simulink model "esm_wanken"  (R2020b)
settings: Solver=FixedStepAuto  StartTime=simin_radius.time(1,1)  StopTime=simin_radius.time(end,1)-0.01  FixedStep=0.01  RelTol=1e-3  EnableMultiTasking=on
values from neighbouring files (symbols this model uses):
  FZGpars =     [Polo_erweitertesESM.mat]
undefined symbols (not defined in the file or in its folder): magnitude
libraries: simulink x8
settings Model: EnablePacing=on  PacingRate=1000  Creator=Administrator  LastModifiedBy=Laptop 11
settings DataIOCC: ExternalInput=[deltal, v]  SaveFormat=Array  SignalLoggingSaveFormat=ModelDataLogs  ReturnWorkspaceOutputs=off
settings OptimizationCC: ExpressionDepthLimit=2147483647  InitFltsAndDblsToZero=on  LifeSpan=inf
settings DebuggingCC: AlgebraicLoopMsg=none  SaveWithParameterizedLinksMsg=none  UnderspecifiedInitializationDetection=Classic  MergeDetectMultiDrivingBlocksExec=none  SignalResolutionControl=TryResolveAllWithWarning  SolverPrmCheckMsg=warning  MultiTaskDSMMsg=warning  MultiTaskCondExecSysMsg=none  FcnCallInpInsideContextMsg=warning  AllowSymbolicDim=off  StateNameClashWarn=warning  SFUnexpectedBacktrackingDiag=warning  SFNoUnconditionalDefaultTransitionDiag=warning  SFExecutionAtInitializationDiag=none  ArithmeticOperatorsInVariantConditions=warning
settings HardwareCC: ProdBitPerPointer=32  ProdBitPerSizeT=32  ProdBitPerPtrDiffT=32  ProdLargestAtomicFloat=None  ProdIntDivRoundTo=Undefined  ProdEndianess=Unspecified  ProdWordSize=32  ProdHWDeviceType=32-bit Generic
settings ModelReferenceCC: PropagateSignalLabelsOutOfModel=off
settings SFSimCC: SimUseLocalCustomCode=off  CustomCodeUndefinedFunction=UseInterfaceOnly
settings RTWCC: RTWUseLocalCustomCode=off
settings CodeAppCC: StateflowObjectComments=on
settings GRTTargetCC: TargetFcnLib=ansi_tfl_tmw.mat  TargetLangStandard=C89/C90 (ANSI)  CombineOutputUpdateFcns=off  GRTInterface=on
settings ConfigComp: CovMetricSettings=dw  CovSaveCumulativeToWorkspaceVar=on  CovSaveSingleToWorkspaceVar=on  CovExternalEMLEnable=off
settings SimscapeCC: SimscapeNormalizeSystem=off
settings ConfigurationSet: Description=SimMechanics 2G

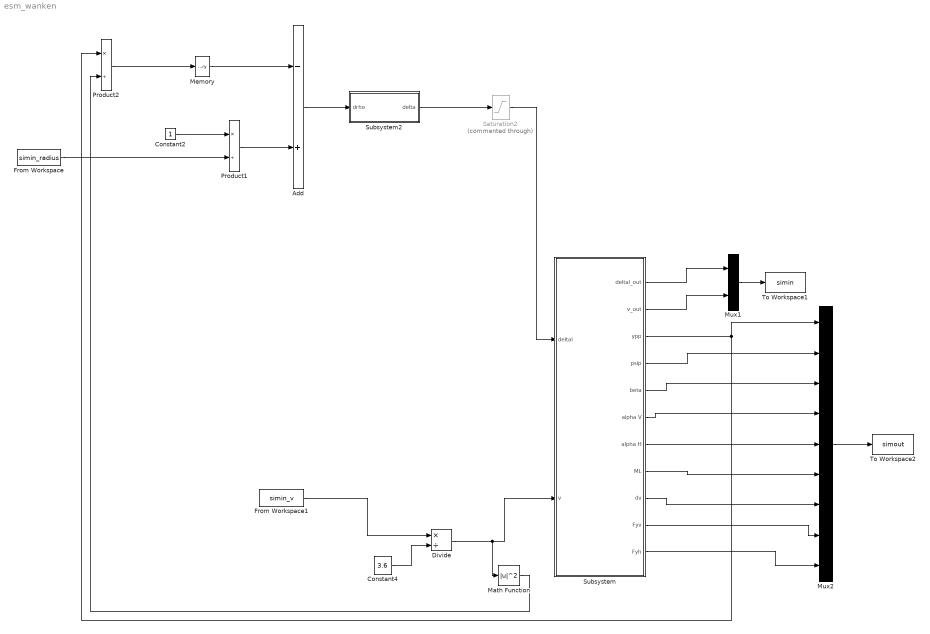
== system esm_wanken ==
  Add : Sum  Inputs=-+
  Constant2 : Constant
  Constant4 : Constant  Value=3.6
  Divide : Product  Inputs=*/
  From Workspace : FromWorkspace  VariableName=simin_radius  OutputAfterFinalValue=Setting to zero
  From Workspace1 : FromWorkspace  VariableName=simin_v  OutputAfterFinalValue=Setting to zero
  Math Function : Math  Operator=magnitude^2  SignedPower=on  SaturateOnIntegerOverflow=on
  Memory : Memory
  Mux1 : Mux  Inputs=2
  Mux2 : Mux  Inputs=9
  Product1 : Product  Inputs=*/  RndMeth=Zero
  Product2 : Product  Inputs=*/  RndMeth=Zero
  Saturation2 : Saturate  Commented=through  UpperLimit=540*pi/180  LowerLimit=-540*pi/180
  Subsystem : Subsystem
  Subsystem2 : Subsystem
  To Workspace1 : ToWorkspace  VariableName=simin  SaveFormat=Structure With Time  SampleTime=-1
  To Workspace2 : ToWorkspace  VariableName=simout  SaveFormat=Structure  SampleTime=-1
  wires:
  Mux1/1 -> To Workspace1/1
  Subsystem/4(psip) -> Mux2/2
  Mux2/1 -> To Workspace2/1
  Subsystem/1(deltal_out) -> Mux1/1
  Subsystem/5(beta) -> Mux2/3
  Subsystem/6(alpha V) -> Mux2/4
  Subsystem/7(alpha H) -> Mux2/5
  Subsystem/2(v_out) -> Mux1/2
  Subsystem/8(ML) -> Mux2/6
  Subsystem/9(dv) -> Mux2/7
  Subsystem/10(Fyv) -> Mux2/8
  Subsystem/11(Fyh) -> Mux2/9
  Subsystem2/1(delta) -> Saturation2/1
  Product1/1 -> Add/2
  Math Function/1 -> Product2/2
  Memory/1 -> Add/1
  Product2/1 -> Memory/1
  Constant2/1 -> Product1/1
  Add/1 -> Subsystem2/1(drho)
  Subsystem/3(ypp) -> Mux2/1, Product2/1
  Saturation2/1 -> Subsystem/1(deltal)
  From Workspace/1 -> Product1/2
  From Workspace1/1 -> Divide/1
  Constant4/1 -> Divide/2
  Divide/1 -> Math Function/1, Subsystem/2(v)

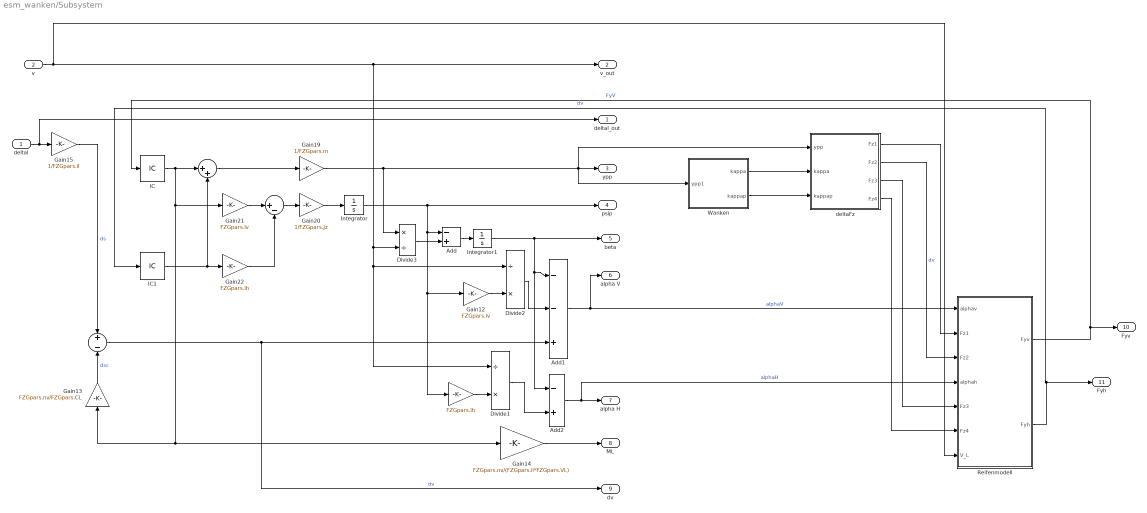
== system esm_wanken/Subsystem ==
  deltal : Inport
  v : Inport  Port=2
  " " : Sum  Inputs=|++
  "  " : Sum  Inputs=|+-
  "   " : Sum  Inputs=+-
  "      " : Gain  Gain=FZGpars.lh
  Add : Sum  Inputs=-+
  Add1 : Sum  Inputs=--+
  Add2 : Sum  Inputs=-+
  Divide1 : Product  Inputs=/*
  Divide2 : Product  Inputs=/*
  Divide3 : Product  Inputs=*/
  Gain12 : Gain  Gain=FZGpars.lv
  Gain13 : Gain  Gain=FZGpars.nv/FZGpars.CL
  Gain14 : Gain  Gain=FZGpars.nv/(FZGpars.il*FZGpars.VL)
  Gain15 : Gain  Gain=1/FZGpars.il
  Gain19 : Gain  Gain=1/FZGpars.m
  Gain20 : Gain  Gain=1/FZGpars.Jz
  Gain21 : Gain  Gain=FZGpars.lv
  Gain22 : Gain  Gain=FZGpars.lh
  IC : InitialCondition
  IC1 : InitialCondition
  Integrator : Integrator
  Integrator1 : Integrator
  Reifenmodell : Subsystem
  Wanken : Subsystem
  deltaFz : Subsystem
  deltal_out : Outport
  v_out : Outport  Port=2
  ypp : Outport  Port=3
  psip : Outport  Port=4
  beta : Outport  Port=5
  alpha V : Outport  Port=6
  alpha H : Outport  Port=7
  ML : Outport  Port=8
  dv : Outport  Port=9
  Fyv : Outport  Port=10
  Fyh : Outport  Port=11
  wires:
  Integrator1/1 -> Add2/1, Add1/1, beta/1
  Divide3/1 -> Add/2
  Integrator/1 -> "      "/1, Gain12/1, Add/1, psip/1
  deltal/1 -> Gain15/1, deltal_out/1
  " "/1 -> Gain19/1
  Gain21/1 -> "  "/1
  Gain22/1 -> "  "/2
  "  "/1 -> Gain20/1
  Gain15/1 -> "   "/1  "ds"
  Gain14/1 -> ML/1
  Add1/1 -> Reifenmodell/1(alphav), alpha V/1  "alphaV"
  Gain20/1 -> Integrator/1
  Add/1 -> Integrator1/1
  "   "/1 -> dv/1, Add1/3  "dv"
  "      "/1 -> Divide1/2
  v/1 -> Reifenmodell/7(V_L), Divide3/2, Divide2/1, Divide1/1, v_out/1
  Divide1/1 -> Add2/2
  Gain12/1 -> Divide2/2
  Divide2/1 -> Add1/2
  Add2/1 -> Reifenmodell/4(alphah), alpha H/1  "alphaH"
  Wanken/1(kappa) -> deltaFz/2(kappa)
  Gain19/1 -> Divide3/1, Wanken/1(ypp1), deltaFz/1(ypp), ypp/1
  Reifenmodell/2(Fyh) -> IC1/1, Fyh/1  "dv"
  deltaFz/1(Fz1) -> Reifenmodell/2("Fz1 ")
  deltaFz/2(Fz2) -> Reifenmodell/3(Fz2)  "dv"
  IC1/1 -> " "/2, Gain22/1
  IC/1 -> " "/1, Gain14/1, Gain13/1, Gain21/1
  Reifenmodell/1(Fyv) -> IC/1, Fyv/1  "FyV"
  Wanken/2("kappap ") -> deltaFz/3("kappap ")
  Gain13/1 -> "   "/2  "dsc"
  deltaFz/3(Fz3) -> Reifenmodell/5(Fz3)
  deltaFz/4(Fz4) -> Reifenmodell/6(Fz4)

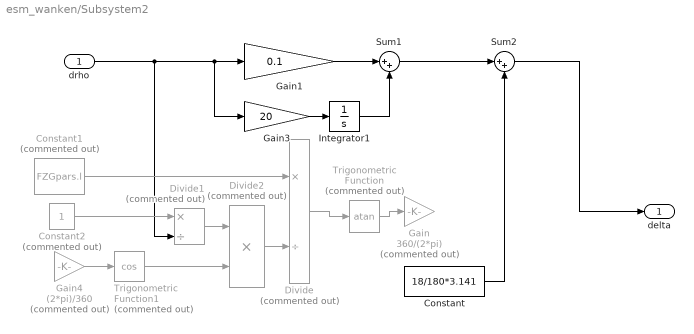
== system esm_wanken/Subsystem2 ==
  drho : Inport
  Constant : Constant  Value=18/180*3.141
  Constant1 : Constant  Commented=on  Value=FZGpars.l
  Constant2 : Constant  Commented=on
  Divide : Product  Commented=on  Inputs=*/
  Divide1 : Product  Commented=on  Inputs=*/
  Divide2 : Product  Commented=on  Inputs=**
  Gain : Gain  Commented=on  Gain=360/(2*pi)
  Gain1 : Gain  Gain=0.1
  Gain3 : Gain  Gain=20
  Gain4 : Gain  Commented=on  Gain=(2*pi)/360
  Integrator1 : Integrator
  Sum1 : Sum  Inputs=|++
  Sum2 : Sum  Inputs=|++
  Trigonometric Function : Trigonometry  Commented=on  Operator=atan  OutputSignalType=real
  Trigonometric Function1 : Trigonometry  Commented=on  Operator=cos  OutputSignalType=real
  delta : Outport
  wires:
  drho/1 -> Gain3/1, Gain1/1, Divide1/2
  Integrator1/1 -> Sum1/2
  Gain1/1 -> Sum1/1
  Gain3/1 -> Integrator1/1
  Constant/1 -> Sum2/2
  Sum1/1 -> Sum2/1
  Constant1/1 -> Divide/1
  Constant2/1 -> Divide1/1
  Divide/1 -> Trigonometric Function/1
  Trigonometric Function/1 -> Gain/1
  Divide1/1 -> Divide2/1
  Divide2/1 -> Divide/2
  Trigonometric Function1/1 -> Divide2/2
  Gain4/1 -> Trigonometric Function1/1
  Sum2/1 -> delta/1

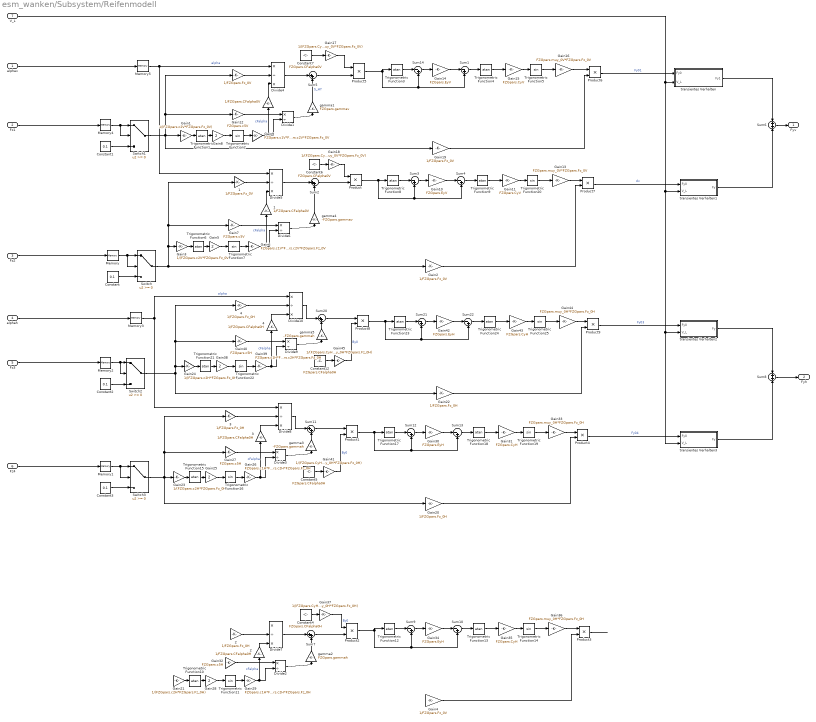
== system esm_wanken/Subsystem/Reifenmodell ==
  alphav : Inport
  "Fz1 " : Inport  Port=2
  Fz2 : Inport  Port=3
  alphah : Inport  Port=4
  Fz3 : Inport  Port=5
  Fz4 : Inport  Port=6
  V_L : Inport  Port=7
  " " : Gain  Gain=1/FZGpars.Fz_0V
  " " : Gain  Gain=1/FZGpars.CFalpha0V
  " 1" : Gain  Gain=1/FZGpars.CFalpha0V
  " 2" : Gain  Gain=1/FZGpars.CFalpha0H
  " 3" : Gain  Gain=1/FZGpars.CFalpha0H
  " 4" : Gain  Gain=1/FZGpars.CFalpha0H
  " 1" : Gain  Gain=1/FZGpars.Fz_0V
  " 2" : Gain  Gain=1/FZGpars.Fz_0H
  " 3" : Gain  Gain=1/FZGpars.Fz_0H
  " 4" : Gain  Gain=1/FZGpars.Fz_0H
  Constant{,1..3} (4 alike) : Constant  Value=0.1
  Constant12 : Constant  Value=FZGpars.CFalpha0H
  Constant4 : Constant  Value=FZGpars.CFalpha0H
  Constant5 : Constant  Value=FZGpars.CFalpha0H
  Constant6 : Constant  Value=FZGpars.CFalpha0V
  Constant7 : Constant  Value=FZGpars.CFalpha0V
  Divide{1..3,6,9} (5 alike) : Product  Inputs=*/
  Divide{4..5,7..8,10} (5 alike) : Product  Inputs=*/*
  Gain1 : Gain  Gain=1/(FZGpars.c2V*FZGpars.Fz_0V)
  Gain10 : Gain  Gain=FZGpars.EyV
  Gain11 : Gain  Gain=FZGpars.CyV
  Gain12 : Gain  Gain=FZGpars.c5V
  Gain13 : Gain  Gain=FZGpars.muy_0V*FZGpars.Fz_0V
  Gain14 : Gain  Gain=FZGpars.EyV
  Gain15 : Gain  Gain=FZGpars.CyV
  Gain16 : Gain  Gain=FZGpars.muy_0V*FZGpars.Fz_0V
  Gain17 : Gain  Gain=1/(FZGpars.CyV*FZGpars.muy_0V*FZGpars.Fz_0V)
  Gain18 : Gain  Gain=1/(FZGpars.CyV*FZGpars.muy_0V*FZGpars.Fz_0V)
  Gain19 : Gain  Gain=1/FZGpars.Fz_0V
  Gain2 : Gain  Gain=1/FZGpars.Fz_0V
  Gain20 : Gain  Gain=1/FZGpars.Fz_0H
  Gain21 : Gain  Gain=1/(FZGpars.c2H*FZGpars.Fz_0H)
  Gain22 : Gain  Gain=1/FZGpars.Fz_0H
  Gain23 : Gain  Gain=1/(FZGpars.c2H*FZGpars.Fz_0H)
  Gain24 : Gain  Gain=1/(FZGpars.c2H*FZGpars.Fz_0H)
  Gain{5,8,25,28,38} (5 alike) : Gain  Gain=2
  Gain26 : Gain  Gain=FZGpars.c1H*FZGpars.c2H*FZGpars.Fz_0H
  Gain27 : Gain  Gain=FZGpars.c5H
  Gain29 : Gain  Gain=FZGpars.c1H*FZGpars.c2H*FZGpars.Fz_0H
  Gain3 : Gain  Gain=1/(FZGpars.c2V*FZGpars.Fz_0V)
  Gain30 : Gain  Gain=FZGpars.EyH
  Gain31 : Gain  Gain=FZGpars.CyH
  Gain32 : Gain  Gain=FZGpars.c5H
  Gain33 : Gain  Gain=FZGpars.muy_0H*FZGpars.Fz_0H
  Gain34 : Gain  Gain=FZGpars.EyH
  Gain35 : Gain  Gain=FZGpars.CyH
  Gain36 : Gain  Gain=FZGpars.muy_0H*FZGpars.Fz_0H
  Gain37 : Gain  Gain=1/(FZGpars.CyH*FZGpars.muy_0H*FZGpars.Fz_0H)
  Gain39 : Gain  Gain=FZGpars.c1H*FZGpars.c2H*FZGpars.Fz_0H
  Gain4 : Gain  Gain=1/FZGpars.Fz_0V
  Gain40 : Gain  Gain=FZGpars.c5H
  Gain41 : Gain  Gain=1/(FZGpars.CyH*FZGpars.muy_0H*FZGpars.Fz_0H)
  Gain42 : Gain  Gain=FZGpars.EyH
  Gain43 : Gain  Gain=FZGpars.CyH
  Gain44 : Gain  Gain=FZGpars.muy_0H*FZGpars.Fz_0H
  Gain45 : Gain  Gain=1/(FZGpars.CyH*FZGpars.muy_0H*FZGpars.Fz_0H)
  Gain6 : Gain  Gain=FZGpars.c1V*FZGpars.c2V*FZGpars.Fz_0V
  Gain7 : Gain  Gain=FZGpars.c5V
  Gain9 : Gain  Gain=FZGpars.c1V*FZGpars.c2V*FZGpars.Fz_0V
  Memory{,1..5} (6 alike) : Memory
  Product{,1..9} (10 alike) : Product
  Sum{1,3..4,9..10,12..14,21..22} (10 alike) : Sum  Inputs=|-+
  Sum{2,5,7,11,20} (5 alike) : Sum  Inputs=|++
  Sum6 : Sum  Inputs=+|+
  Sum8 : Sum  Inputs=+|+
  Switch{,1..3} (4 alike) : Switch
  Trigonometric Function{1,3..4,6,8..10,12..13,15,17..18,21,23..24} (15 alike) : Trigonometry  Operator=atan
  Trigonometric Function{2,5,7,11,14,16,19..20,22,25} (10 alike) : Trigonometry
  gamma1 : Gain  Gain=FZGpars.gammav
  gamma2 : Gain  Gain=FZGpars.gammah
  gamma3 : Gain  Gain=-FZGpars.gammah
  gamma4 : Gain  Gain=-FZGpars.gammav
  gamma5 : Gain  Gain=-FZGpars.gammah
  transientes Verhalten : Subsystem
  transientes Verhalten1 : Subsystem
  transientes Verhalten2 : Subsystem
  transientes Verhalten3 : Subsystem
  Fyv : Outport
  Fyh : Outport  Port=2
  wires:
  Gain23/1 -> Trigonometric Function15/1
  Trigonometric Function15/1 -> Gain25/1
  Gain25/1 -> Trigonometric Function16/1
  Trigonometric Function16/1 -> Gain26/1
  gamma3/1 -> Sum11/2
  Divide3/1 -> gamma3/1
  Product1/1 -> Sum13/2, Sum12/2, Trigonometric Function17/1
  Trigonometric Function17/1 -> Sum12/1
  Sum12/1 -> Gain30/1
  Gain30/1 -> Sum13/1
  Sum13/1 -> Trigonometric Function18/1
  Trigonometric Function18/1 -> Gain31/1
  Gain31/1 -> Trigonometric Function19/1
  Trigonometric Function19/1 -> Gain33/1
  Gain33/1 -> Product4/1
  Gain27/1 -> Divide3/1
  Gain41/1 -> Product1/2  "By0"
  Sum11/1 -> Product1/1
  Sum6/1 -> Fyv/1
  Memory5/1 -> Divide5/1, Divide4/1  "alpha"
  Gain3/1 -> Trigonometric Function6/1
  Trigonometric Function6/1 -> Gain5/1
  Gain5/1 -> Trigonometric Function7/1
  Trigonometric Function7/1 -> Gain6/1
  gamma4/1 -> Sum2/2
  Divide6/1 -> gamma4/1
  Product/1 -> Sum4/2, Sum3/2, Trigonometric Function8/1
  Trigonometric Function8/1 -> Sum3/1
  Sum3/1 -> Gain10/1
  Gain10/1 -> Sum4/1
  Sum4/1 -> Trigonometric Function9/1
  Trigonometric Function9/1 -> Gain11/1
  Gain11/1 -> Trigonometric Function20/1
  Trigonometric Function20/1 -> Gain13/1
  Gain13/1 -> Product7/1
  Gain7/1 -> Divide6/1
  Gain18/1 -> Product/1
  Sum2/1 -> Product/2
  Gain1/1 -> Trigonometric Function1/1
  Trigonometric Function1/1 -> Gain8/1
  Gain8/1 -> Trigonometric Function2/1
  Trigonometric Function2/1 -> Gain9/1
  Gain9/1 -> " "/1, Divide1/2  "cFalpha"
  gamma1/1 -> Sum5/2  "S_HY"
  Divide1/1 -> gamma1/1
  Product5/1 -> Trigonometric Function3/1, Sum1/2, Sum14/2
  Trigonometric Function3/1 -> Sum14/1
  Sum14/1 -> Gain14/1
  Gain14/1 -> Sum1/1
  Sum1/1 -> Trigonometric Function4/1
  Trigonometric Function4/1 -> Gain15/1
  Gain15/1 -> Trigonometric Function5/1
  Trigonometric Function5/1 -> Gain16/1
  Gain16/1 -> Product6/1
  Gain12/1 -> Divide1/1
  Gain17/1 -> Product5/1
  Switch1/1 -> " "/1, Gain12/1, Gain19/1, Gain1/1
  Switch/1 -> Gain2/1, " 1"/1, Gain7/1, Gain3/1
  Gain20/1 -> Product4/2
  alphav/1 -> Memory5/1
  Memory/1 -> Switch/1, Switch/2
  Constant/1 -> Switch/3
  Memory4/1 -> Switch1/2, Switch1/1
  Constant1/1 -> Switch1/3
  Memory2/1 -> Switch2/2, Switch2/1
  Constant2/1 -> Switch2/3
  Memory1/1 -> Switch3/2, Switch3/1
  Constant3/1 -> Switch3/3
  transientes Verhalten/1(Fy1) -> Sum6/1
  transientes Verhalten1/1(Fy) -> Sum6/2
  V_L/1 -> transientes Verhalten1/2(V_L), transientes Verhalten2/2(V_L), transientes Verhalten3/2(V_L), transientes Verhalten/2(V_L)
  Divide4/1 -> Sum5/1
  " "/1 -> Divide4/3
  " "/1 -> Divide4/2
  Gain6/1 -> " 1"/1, Divide6/2  "cFalpha"
  " 1"/1 -> Divide5/3
  Divide5/1 -> Sum2/1
  " 1"/1 -> Divide5/2
  Memory3/1 -> Divide8/1, Divide10/1  "alpha"
  Gain26/1 -> " 3"/1, Divide3/2  "cFalpha"
  Switch3/1 -> Gain20/1, " 3"/1, Gain27/1, Gain23/1
  Divide8/1 -> Sum11/1
  " 3"/1 -> Divide8/3
  " 3"/1 -> Divide8/2
  Constant5/1 -> Gain41/1
  Constant6/1 -> Gain18/1
  Constant7/1 -> Gain17/1
  Sum5/1 -> Product5/2
  Gain19/1 -> Product6/2
  Gain2/1 -> Product7/2
  transientes Verhalten2/1(Fy) -> Sum8/1
  transientes Verhalten3/1(Fy) -> Sum8/2
  "Fz1 "/1 -> Memory4/1
  Fz2/1 -> Memory/1
  alphah/1 -> Memory3/1
  Fz3/1 -> Memory2/1
  Fz4/1 -> Memory1/1
  Gain21/1 -> Trigonometric Function10/1
  Trigonometric Function10/1 -> Gain28/1
  Gain28/1 -> Trigonometric Function11/1
  Trigonometric Function11/1 -> Gain29/1
  gamma2/1 -> Sum7/2
  Divide2/1 -> gamma2/1
  Product2/1 -> Trigonometric Function12/1, Sum10/2, Sum9/2
  Trigonometric Function12/1 -> Sum9/1
  Sum9/1 -> Gain34/1
  Gain34/1 -> Sum10/1
  Sum10/1 -> Trigonometric Function13/1
  Trigonometric Function13/1 -> Gain35/1
  Gain35/1 -> Trigonometric Function14/1
  Trigonometric Function14/1 -> Gain36/1
  Gain36/1 -> Product3/1
  Gain32/1 -> Divide2/1
  Gain37/1 -> Product2/1  "By0"
  Gain4/1 -> Product3/2
  Product3/1 -> ?
  ? -> Divide7/1  "alpha"
  Gain29/1 -> " 2"/1, Divide2/2  "cFalpha"
  ? -> Gain4/1, " 2"/1, Gain32/1, Gain21/1
  Divide7/1 -> Sum7/1
  " 2"/1 -> Divide7/3
  " 2"/1 -> Divide7/2
  Constant4/1 -> Gain37/1
  Sum7/1 -> Product2/2
  Gain24/1 -> Trigonometric Function21/1
  Trigonometric Function21/1 -> Gain38/1
  Gain38/1 -> Trigonometric Function22/1
  Trigonometric Function22/1 -> Gain39/1
  gamma5/1 -> Sum20/2
  Divide9/1 -> gamma5/1
  Product8/1 -> Sum22/2, Sum21/2, Trigonometric Function23/1
  Trigonometric Function23/1 -> Sum21/1
  Sum21/1 -> Gain42/1
  Gain42/1 -> Sum22/1
  Sum22/1 -> Trigonometric Function24/1
  Trigonometric Function24/1 -> Gain43/1
  Gain43/1 -> Trigonometric Function25/1
  Trigonometric Function25/1 -> Gain44/1
  Gain44/1 -> Product9/1
  Gain40/1 -> Divide9/1
  Gain45/1 -> Product8/2  "By0"
  Sum20/1 -> Product8/1
  Gain22/1 -> Product9/2
  Gain39/1 -> " 4"/1, Divide9/2  "cFalpha"
  Switch2/1 -> " 4"/1, Gain40/1, Gain24/1, Gain22/1
  Divide10/1 -> Sum20/1
  " 4"/1 -> Divide10/3
  " 4"/1 -> Divide10/2
  Constant12/1 -> Gain45/1
  Product6/1 -> transientes Verhalten/1(Fy0)  "Fy01"
  Product9/1 -> transientes Verhalten2/1(Fy0)  "Fy03"
  Product4/1 -> transientes Verhalten3/1(Fy0)  "Fy04"
  Sum8/1 -> Fyh/1
  Product7/1 -> transientes Verhalten1/1(Fy0)  "dv"

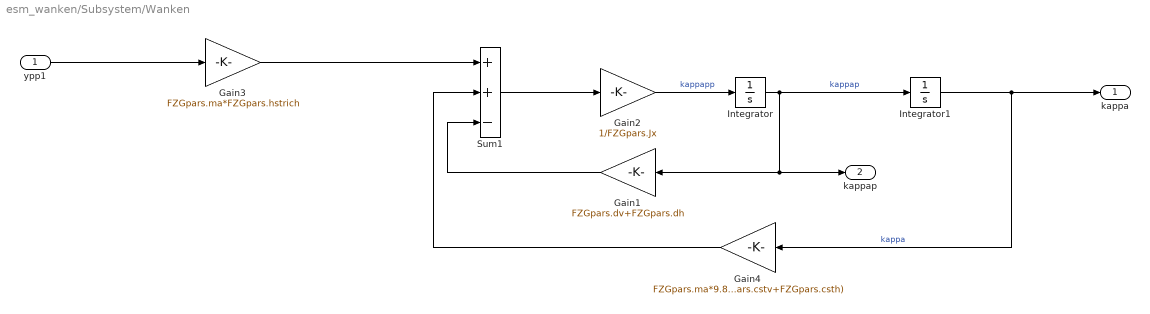
== system esm_wanken/Subsystem/Wanken ==
  ypp1 : Inport
  Gain1 : Gain  Gain=FZGpars.dv+FZGpars.dh
  Gain2 : Gain  Gain=1/FZGpars.Jx
  Gain3 : Gain  Gain=FZGpars.ma*FZGpars.hstrich
  Gain4 : Gain  Gain=FZGpars.ma*9.81*FZGpars.hstrich-(FZGpars.cv+FZGpars.ch+FZGpars.cstv+FZGpars.csth)
  Integrator : Integrator
  Integrator1 : Integrator
  Sum1 : Sum  Inputs=++-
  kappa : Outport
  "kappap " : Outport  Port=2
  wires:
  Gain2/1 -> Integrator/1  "kappapp"
  Gain3/1 -> Sum1/1
  Gain4/1 -> Sum1/2
  Gain1/1 -> Sum1/3
  Sum1/1 -> Gain2/1
  ypp1/1 -> Gain3/1
  Integrator/1 -> Integrator1/1, "kappap "/1, Gain1/1  "kappap"
  Integrator1/1 -> kappa/1, Gain4/1  "kappa"

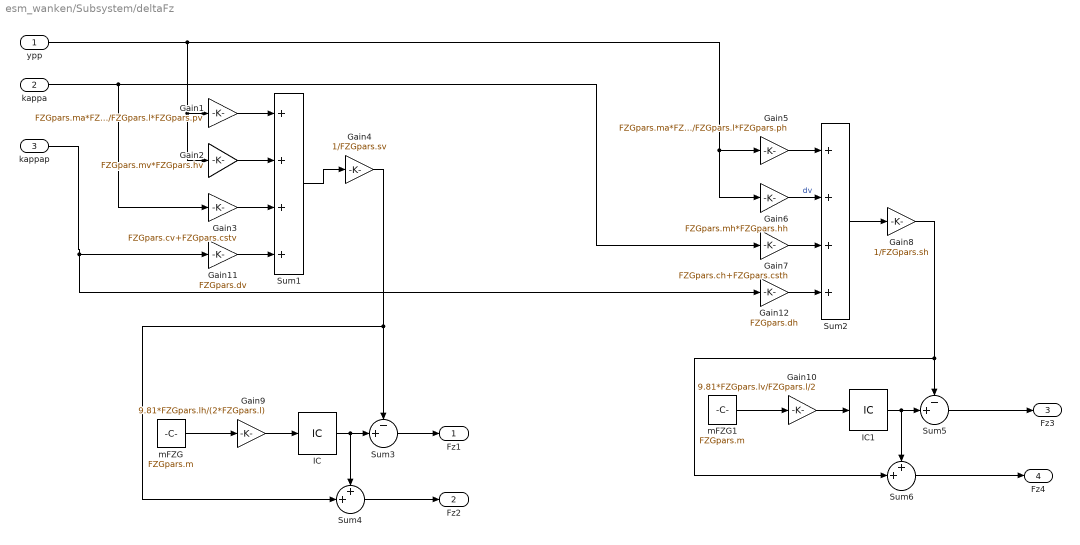
== system esm_wanken/Subsystem/deltaFz ==
  ypp : Inport
  kappa : Inport  Port=2
  "kappap " : Inport  Port=3
  Gain1 : Gain  Gain=FZGpars.ma*FZGpars.lh/FZGpars.l*FZGpars.pv
  Gain10 : Gain  Gain=9.81*FZGpars.lv/FZGpars.l/2
  Gain11 : Gain  Gain=FZGpars.dv
  Gain12 : Gain  Gain=FZGpars.dh
  Gain2 : Gain  Gain=FZGpars.mv*FZGpars.hv
  Gain3 : Gain  Gain=FZGpars.cv+FZGpars.cstv
  Gain4 : Gain  Gain=1/FZGpars.sv
  Gain5 : Gain  Gain=FZGpars.ma*FZGpars.lv/FZGpars.l*FZGpars.ph
  Gain6 : Gain  Gain=FZGpars.mh*FZGpars.hh
  Gain7 : Gain  Gain=FZGpars.ch+FZGpars.csth
  Gain8 : Gain  Gain=1/FZGpars.sh
  Gain9 : Gain  Gain=9.81*FZGpars.lh/(2*FZGpars.l)
  IC : InitialCondition  Value=FZGpars.m*(9.81*FZGpars.lh/(2*FZGpars.l))
  IC1 : InitialCondition  Value=FZGpars.m*(9.81*FZGpars.lv/FZGpars.l/2)
  Sum1 : Sum  Inputs=++++
  Sum2 : Sum  Inputs=++++
  Sum3 : Sum  Inputs=-+|
  Sum4 : Sum  Inputs=++|
  Sum5 : Sum  Inputs=-+|
  Sum6 : Sum  Inputs=++|
  mFZG : Constant  Value=FZGpars.m
  mFZG1 : Constant  Value=FZGpars.m
  Fz1 : Outport
  Fz2 : Outport  Port=2
  Fz3 : Outport  Port=3
  Fz4 : Outport  Port=4
  wires:
  Gain2/1 -> Sum1/2
  Gain1/1 -> Sum1/1
  Gain3/1 -> Sum1/3
  Sum1/1 -> Gain4/1
  Gain5/1 -> Sum2/1
  Sum2/1 -> Gain8/1
  mFZG/1 -> Gain9/1
  Gain9/1 -> IC/1
  mFZG1/1 -> Gain10/1
  Gain10/1 -> IC1/1
  Sum3/1 -> Fz1/1
  Sum4/1 -> Fz2/1
  Sum5/1 -> Fz3/1
  Sum6/1 -> Fz4/1
  Gain4/1 -> Sum4/2, Sum3/1
  Gain8/1 -> Sum6/2, Sum5/1
  kappa/1 -> Gain3/1, Gain7/1
  "kappap "/1 -> Gain12/1, Gain11/1
  Gain11/1 -> Sum1/4
  Gain7/1 -> Sum2/3
  Gain12/1 -> Sum2/4
  ypp/1 -> Gain6/1, Gain5/1, Gain2/1, Gain1/1
  Gain6/1 -> Sum2/2  "dv"
  IC/1 -> Sum4/1, Sum3/2
  IC1/1 -> Sum6/1, Sum5/2

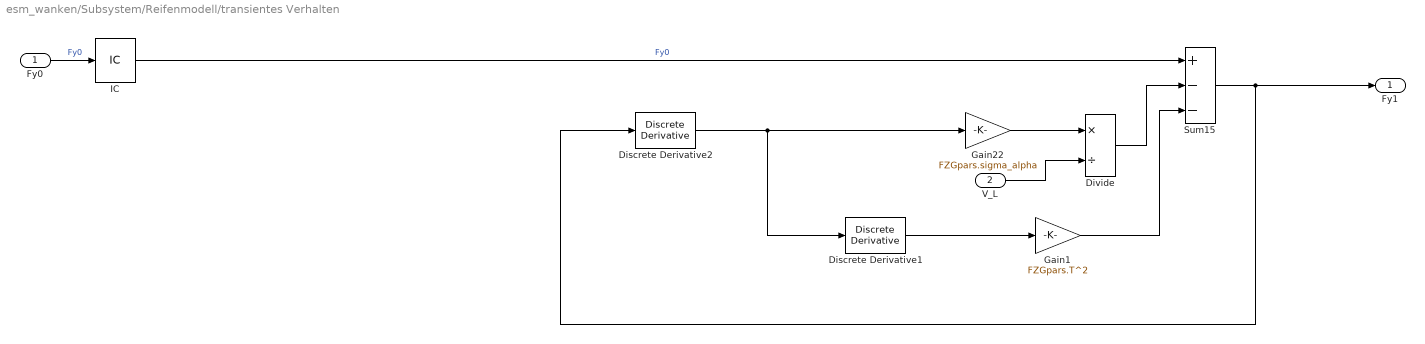
== system esm_wanken/Subsystem/Reifenmodell/transientes Verhalten ==
  Fy0 : Inport
  V_L : Inport  Port=2
  Discrete Derivative1 : simulink/Discrete/Discrete Derivative  gainval=1.0  ICPrevScaledInput=0.0  OutMin=[]  OutMax=[]  OutDataType=fixdt(1, 16)  OutScaling=2^-10  DoSatur=off
  Discrete Derivative2 : simulink/Discrete/Discrete Derivative  gainval=1.0  ICPrevScaledInput=0.0  OutMin=[]  OutMax=[]  OutDataType=fixdt(1, 16)  OutScaling=2^-10  DoSatur=off
  Divide : Product  Inputs=*/
  Gain1 : Gain  Gain=FZGpars.T^2
  Gain22 : Gain  Gain=FZGpars.sigma_alpha
  IC : InitialCondition
  Sum15 : Sum  Inputs=+--
  Fy1 : Outport
  wires:
  Fy0/1 -> IC/1  "Fy0"
  Divide/1 -> Sum15/2
  Gain22/1 -> Divide/1
  V_L/1 -> Divide/2
  Gain1/1 -> Sum15/3
  Discrete Derivative1/1 -> Gain1/1
  IC/1 -> Sum15/1  "Fy0"
  Sum15/1 -> Discrete Derivative2/1, Fy1/1
  Discrete Derivative2/1 -> Discrete Derivative1/1, Gain22/1

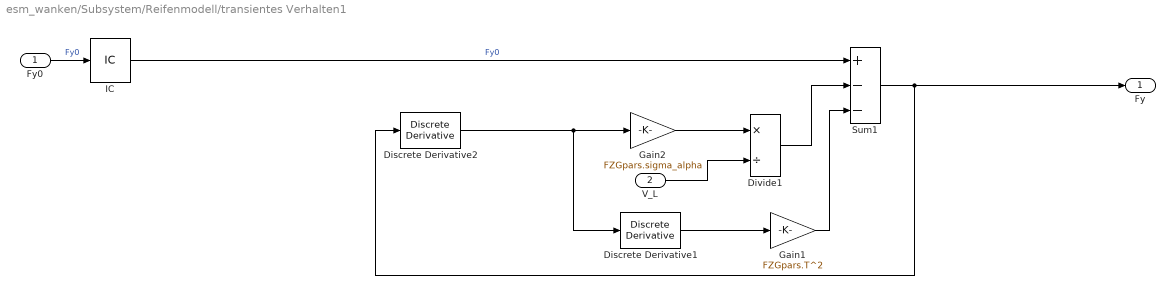
== system esm_wanken/Subsystem/Reifenmodell/transientes Verhalten1 ==
  Fy0 : Inport
  V_L : Inport  Port=2
  Discrete Derivative1 : simulink/Discrete/Discrete Derivative  gainval=1.0  ICPrevScaledInput=0.0  OutMin=[]  OutMax=[]  OutDataType=fixdt(1, 16)  OutScaling=2^-10  DoSatur=off
  Discrete Derivative2 : simulink/Discrete/Discrete Derivative  gainval=1.0  ICPrevScaledInput=0.0  OutMin=[]  OutMax=[]  OutDataType=fixdt(1, 16)  OutScaling=2^-10  DoSatur=off
  Divide1 : Product  Inputs=*/
  Gain1 : Gain  Gain=FZGpars.T^2
  Gain2 : Gain  Gain=FZGpars.sigma_alpha
  IC : InitialCondition
  Sum1 : Sum  Inputs=+--
  Fy : Outport
  wires:
  Fy0/1 -> IC/1  "Fy0"
  Divide1/1 -> Sum1/2
  Gain2/1 -> Divide1/1
  V_L/1 -> Divide1/2
  Gain1/1 -> Sum1/3
  Discrete Derivative1/1 -> Gain1/1
  IC/1 -> Sum1/1  "Fy0"
  Discrete Derivative2/1 -> Discrete Derivative1/1, Gain2/1
  Sum1/1 -> Fy/1, Discrete Derivative2/1

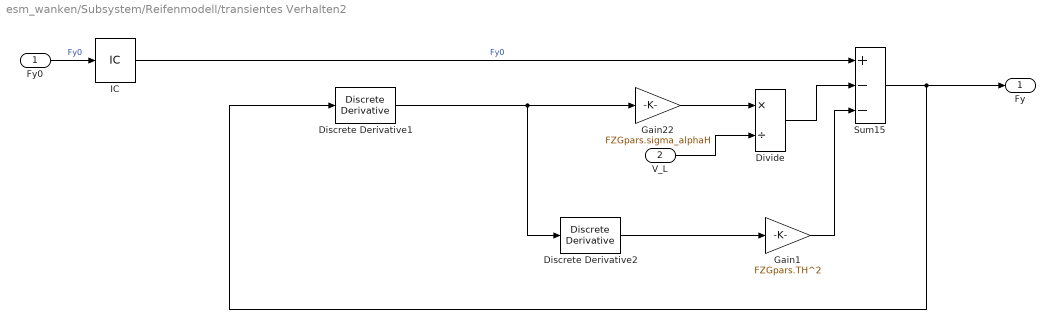
== system esm_wanken/Subsystem/Reifenmodell/transientes Verhalten2 ==
  Fy0 : Inport
  V_L : Inport  Port=2
  Discrete Derivative1 : simulink/Discrete/Discrete Derivative  gainval=1.0  ICPrevScaledInput=0.0  OutMin=[]  OutMax=[]  OutDataType=fixdt(1, 16)  OutScaling=2^-10  DoSatur=off
  Discrete Derivative2 : simulink/Discrete/Discrete Derivative  gainval=1.0  ICPrevScaledInput=0.0  OutMin=[]  OutMax=[]  OutDataType=fixdt(1, 16)  OutScaling=2^-10  DoSatur=off
  Divide : Product  Inputs=*/
  Gain1 : Gain  Gain=FZGpars.TH^2
  Gain22 : Gain  Gain=FZGpars.sigma_alphaH
  IC : InitialCondition
  Sum15 : Sum  Inputs=+--
  Fy : Outport
  wires:
  Fy0/1 -> IC/1  "Fy0"
  Divide/1 -> Sum15/2
  Gain22/1 -> Divide/1
  V_L/1 -> Divide/2
  Gain1/1 -> Sum15/3
  Discrete Derivative2/1 -> Gain1/1
  Sum15/1 -> Discrete Derivative1/1, Fy/1
  IC/1 -> Sum15/1  "Fy0"
  Discrete Derivative1/1 -> Discrete Derivative2/1, Gain22/1

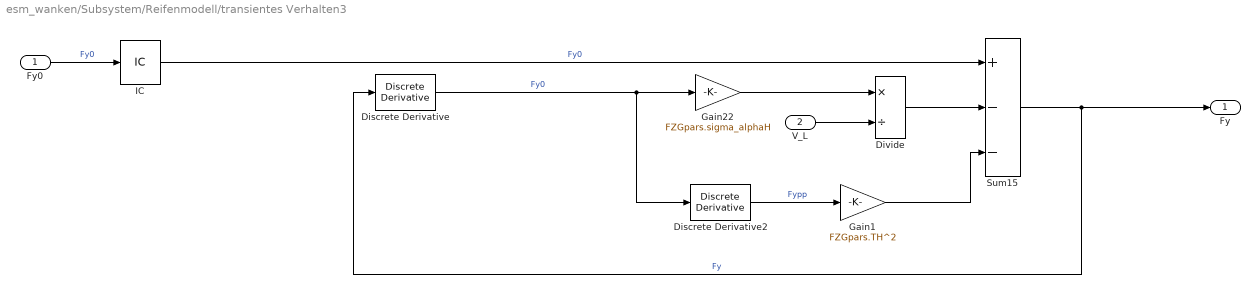
== system esm_wanken/Subsystem/Reifenmodell/transientes Verhalten3 ==
  Fy0 : Inport
  V_L : Inport  Port=2
  Discrete Derivative : simulink/Discrete/Discrete Derivative  gainval=1.0  ICPrevScaledInput=0.0  OutMin=[]  OutMax=[]  OutDataType=fixdt(1, 16)  OutScaling=2^-10  DoSatur=off
  Discrete Derivative2 : simulink/Discrete/Discrete Derivative  gainval=1.0  ICPrevScaledInput=0.0  OutMin=[]  OutMax=[]  OutDataType=fixdt(1, 16)  OutScaling=2^-10  DoSatur=off
  Divide : Product  Inputs=*/
  Gain1 : Gain  Gain=FZGpars.TH^2
  Gain22 : Gain  Gain=FZGpars.sigma_alphaH
  IC : InitialCondition
  Sum15 : Sum  Inputs=+--
  Fy : Outport
  wires:
  Gain22/1 -> Divide/1
  Fy0/1 -> IC/1  "Fy0"
  Sum15/1 -> Discrete Derivative/1, Fy/1  "Fy"
  IC/1 -> Sum15/1  "Fy0"
  Discrete Derivative2/1 -> Gain1/1  "Fypp"
  Divide/1 -> Sum15/2
  Gain1/1 -> Sum15/3
  Discrete Derivative/1 -> Discrete Derivative2/1, Gain22/1  "Fy0"
  V_L/1 -> Divide/2
